simulink model "subsys"  (R2014b)
settings: Solver=ode45  StartTime=0.0  StopTime=10.0  RelTol=1e-3
settings Model: Creator=ravoson  LastModifiedBy=ravoson

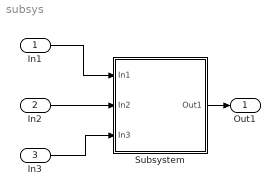
== system subsys ==
  In1 : Inport
  In2 : Inport  Port=2
  In3 : Inport  Port=3
  Subsystem : Subsystem
  Out1 : Outport
  wires:
  In1/1 -> Subsystem/1(In1)
  In2/1 -> Subsystem/2(In2)
  Subsystem/1(Out1) -> Out1/1
  In3/1 -> Subsystem/3(In3)

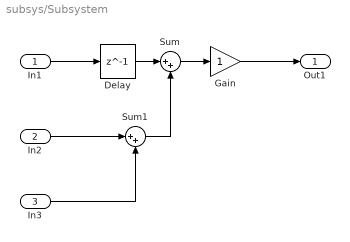
== system subsys/Subsystem ==
  In1 : Inport
  In2 : Inport  Port=2
  In3 : Inport  Port=3
  Delay : Delay  DelayLength=1  InitialCondition=0
  Gain : Gain
  Sum : Sum  Inputs=|++
  Sum1 : Sum  Inputs=|++
  Out1 : Outport
  wires:
  Delay/1 -> Sum/1
  Gain/1 -> Out1/1
  Sum/1 -> Gain/1
  In1/1 -> Delay/1
  In2/1 -> Sum1/1
  In3/1 -> Sum1/2
  Sum1/1 -> Sum/2
